simulink model "rlc_simulinkFinish"  (R2014a)
settings: Solver=ode45  StartTime=0.0  StopTime=1  MaxStep=0.01  RelTol=1e-4
PreLoadFcn:
  | Vs = 30;
  | L = 1e-3;
  | C = 1e-3;
  | R = 1;
settings Model: Creator=cosorio  LastModifiedBy=cosorio

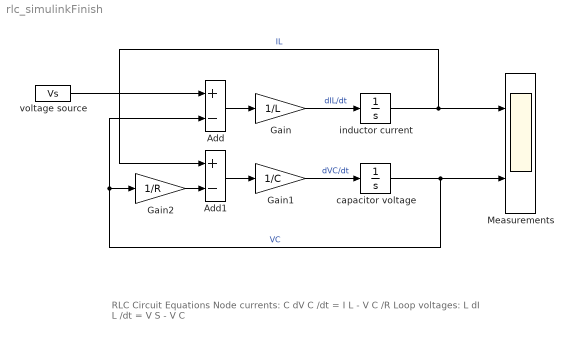
== system rlc_simulinkFinish ==
  note: RLC Circuit Equations
      |
      | Node currents: C dV C /dt = I L - V C /R
      |
      | Loop voltages: L dI L /dt = V S - V C
  Add : Sum  Inputs=+-
  Add1 : Sum  Inputs=+-
  Gain : Gain  Gain=1/L
  Gain1 : Gain  Gain=1/C
  Gain2 : Gain  Gain=1/R
  Measurements : Scope  NumInputPorts=2
      settings: YMin=0~0  YMax=40~40
  capacitor voltage : Integrator
  inductor current : Integrator
  voltage source : Constant  Value=Vs
  wires:
  Gain/1 -> inductor current/1  "dIL/dt"
  inductor current/1 -> Add1/1, Measurements/1  "IL"
  Gain1/1 -> capacitor voltage/1  "dVC/dt"
  capacitor voltage/1 -> Gain2/1, Add/2, Measurements/2  "VC"
  voltage source/1 -> Add/1
  Add/1 -> Gain/1
  Add1/1 -> Gain1/1
  Gain2/1 -> Add1/2
